simulink library "EnergyMeter"  (R2018b)
settings: Solver=ode45  StartTime=0.0  StopTime=10.0  RelTol=1e-3  EnableMultiTasking=on
libraries: carnot x1
settings Model: Creator=lena.frank  LastModifiedBy=P41573
settings DataIOCC: LimitDataPoints=on  SaveFormat=Array  SignalLoggingSaveFormat=ModelDataLogs
settings OptimizationCC: ExpressionDepthLimit=2147483647  LifeSpan=inf
settings DebuggingCC: UnderspecifiedInitializationDetection=Classic  MergeDetectMultiDrivingBlocksExec=none  SolverPrmCheckMsg=warning  FcnCallInpInsideContextMsg=warning  StateNameClashWarn=warning  SFUnexpectedBacktrackingDiag=warning  SFNoUnconditionalDefaultTransitionDiag=warning  SFExecutionAtInitializationDiag=none
settings HardwareCC: ProdBitPerPointer=32  ProdBitPerSizeT=32  ProdBitPerPtrDiffT=32  ProdLargestAtomicFloat=None  ProdIntDivRoundTo=Undefined  ProdEndianess=Unspecified  ProdWordSize=32  ProdHWDeviceType=32-bit Generic
settings ModelReferenceCC: PropagateSignalLabelsOutOfModel=off
settings SFSimCC: SimUseLocalCustomCode=off
settings RTWCC: RTWUseLocalCustomCode=off
settings CodeAppCC: StateflowObjectComments=on
settings GRTTargetCC: TargetLangStandard=C89/C90 (ANSI)  GeneratePreprocessorConditionals=Disable all  CombineOutputUpdateFcns=off  GRTInterface=on
settings ConfigComp: CovMetricSettings=dw  CovHtmlReporting=on  CovSaveCumulativeToWorkspaceVar=on  CovSaveSingleToWorkspaceVar=on  CovExternalEMLEnable=off

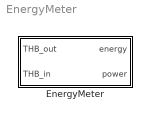
== system EnergyMeter ==
  EnergyMeter : Subsystem  mask(energy meter){}
      mask help: Calculates the power and energy of a fluid flow between inlet and outlet of components.
      mask Help: web(fullfile(path_carnot('help'),'EnergyMeter.html'),'-helpbrowser')

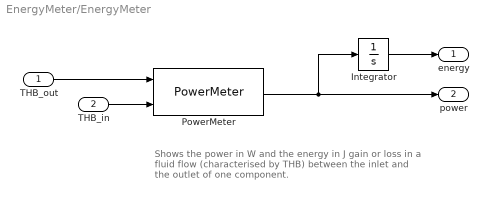
== system EnergyMeter/EnergyMeter ==
  note: Shows the power in W and the energy in J gain or loss
      | in a fluid flow (characterised by THB) between the
      | inlet and the outlet of one component.
  THB_out : Inport
  THB_in : Inport  Port=2
  Integrator : Integrator  UpperSaturationLimit=1  LowerSaturationLimit=0
  PowerMeter : carnot/Control/PowerMeter
      settings: SourceProductName=Carnot
  energy : Outport
  power : Outport  Port=2
  wires:
  PowerMeter/1 -> Integrator/1, power/1
  THB_in/1 -> PowerMeter/2
  Integrator/1 -> energy/1
  THB_out/1 -> PowerMeter/1
